simulink model "NAV420_Emulator"  (Simulink 7.3)
settings: Solver=ode45  StartTime=0.0  StopTime=inf  RelTol=1e-3
undefined symbols (not defined in the file or in its folder): serial
libraries: instrumentlib x2
settings Model: Creator=djulzz  LastModifiedBy=djulzz

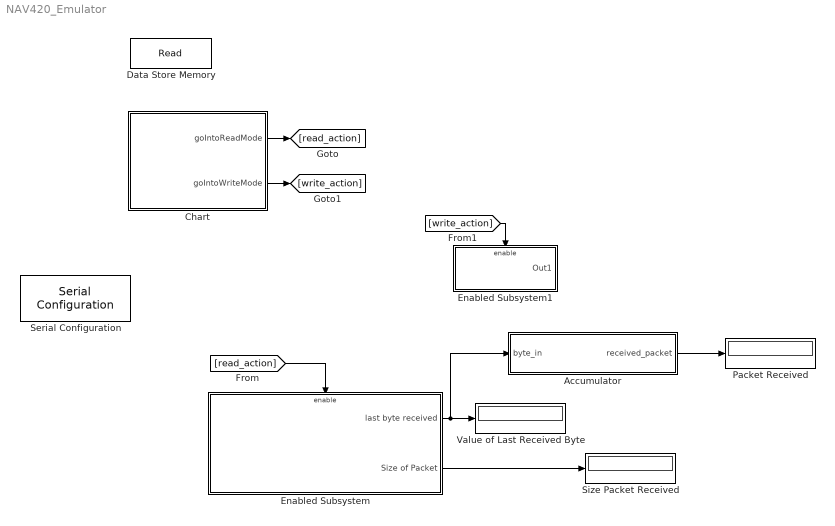
== system NAV420_Emulator ==
  Accumulator : Subsystem
  Chart : Stateflow chart
  Data Store Memory : DataStoreMemory  DataStoreName=Read  ReadBeforeWriteMsg=warning  WriteAfterWriteMsg=warning  WriteAfterReadMsg=warning  InitialValue=1  DataType=double  OutDataType=fixdt(1, 16)  OutScaling=2^0  OutDataTypeStr=double
  Enabled Subsystem : Subsystem  TreatAsAtomicUnit=on
  Enabled Subsystem1 : Subsystem  TreatAsAtomicUnit=on
  Packet Received : Display
  Serial Configuration : instrumentlib/Serial Configuration  Priority=-200000  DialogController=instrumentcreatedialog  DialogControllerArgs=DataTag1  ComPortMenu=COM1  ComPort=COM1  ObjConstructor=serial('COM1');  BaudRate=9600  DataBits=8  Parity=none  StopBits=1  FlowControl=none  Timeout=10  ByteOrder=LittleEndian
  Size Packet Received : Display
  Value of Last Received Byte : Display
  wires:
  Chart/1(goIntoReadMode) -> [read_action]
  Chart/2(goIntoWriteMode) -> [write_action]
  [write_action] -> Enabled Subsystem1/Enable
  Enabled Subsystem/1(last byte received) -> Value of Last Received Byte/1, Accumulator/1(byte_in)
  Enabled Subsystem/2(Size of Packet) -> Size Packet Received/1
  [read_action] -> Enabled Subsystem/Enable
  Accumulator/1(received_packet) -> Packet Received/1

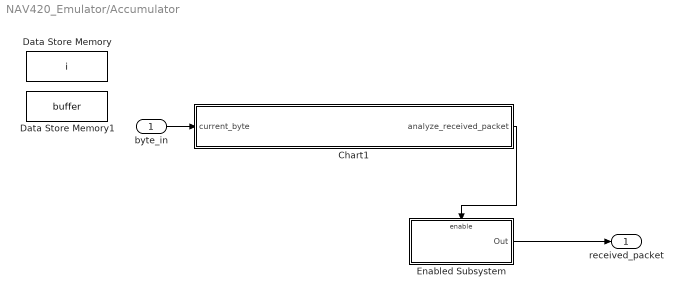
== system NAV420_Emulator/Accumulator ==
  byte_in : Inport  DataType=uint8  OutDataType=fixdt(1, 16)  OutScaling=2^0  OutDataTypeStr=uint8
  Chart1 : Stateflow chart
  Data Store Memory : DataStoreMemory  DataStoreName=i  InitialValue=1  DataType=uint8  OutDataType=fixdt(1, 16)  OutScaling=2^0  OutDataTypeStr=uint8
  Data Store Memory1 : DataStoreMemory  DataStoreName=buffer  InitialValue=1  DataType=uint8  OutDataType=fixdt(1, 16)  OutScaling=2^0  OutDataTypeStr=uint8
  Enabled Subsystem : Subsystem  TreatAsAtomicUnit=on
  received_packet : Outport  DataType=uint8  OutDataType=fixdt(1, 16)  OutScaling=2^0  OutDataTypeStr=uint8
  wires:
  byte_in/1 -> Chart1/1(current_byte)
  Enabled Subsystem/1(Out) -> received_packet/1
  Chart1/1(analyze_received_packet) -> Enabled Subsystem/Enable

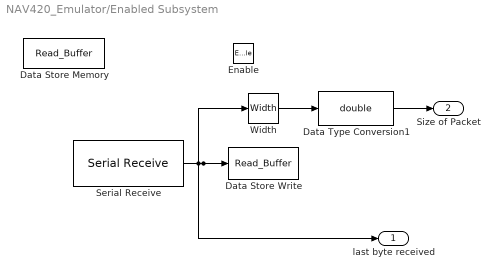
== system NAV420_Emulator/Enabled Subsystem ==
  Enable : EnablePort
  Data Store Memory : DataStoreMemory  DataStoreName=Read_Buffer  InitialValue=1  DataType=uint8  OutDataType=fixdt(1, 16)  OutScaling=2^0  OutDataTypeStr=uint8
  Data Store Write : DataStoreWrite  DataStoreName=Read_Buffer  SampleTime=-1
  Data Type Conversion1 : DataTypeConversion  OutDataTypeMode=double  OutDataType=fixdt(1, 16)  OutScaling=2^0  OutDataTypeStr=double
  Serial Receive : instrumentlib/Serial Receive  DialogController=instrumentcreatedialog  DialogControllerArgs=DataTag0  ComPortMenu=COM1  ComPort=COM1  ObjConstructor=serial('COM1');  Terminator=<none>  DataSize="[1  1]"  DataType=uint8  EnableBlockingMode=on  ActionDataUnavailable=Output last received value  CustomValue=0  SampleTime=0.01
  Width : Width
  last byte received : Outport  DataType=uint8  OutDataType=fixdt(1, 16)  OutScaling=2^0  OutDataTypeStr=uint8
  Size of Packet : Outport  Port=2  DataType=double  OutDataType=fixdt(1, 16)  OutScaling=2^0  OutDataTypeStr=double
  wires:
  Serial Receive/1 -> Data Store Write/1, Width/1, last byte received/1
  Data Type Conversion1/1 -> Size of Packet/1
  Width/1 -> Data Type Conversion1/1

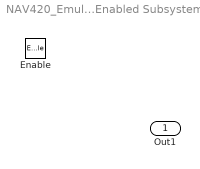
== system NAV420_Emulator/Enabled Subsystem1 ==
  Enable : EnablePort
  Out1 : Outport  OutDataType=fixdt(1, 16)  OutScaling=2^0

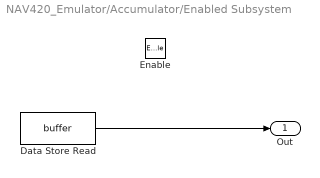
== system NAV420_Emulator/Accumulator/Enabled Subsystem ==
  Enable : EnablePort
  Data Store Read : DataStoreRead  DataStoreName=buffer  SampleTime=0
  Out : Outport  OutDataType=fixdt(1, 16)  OutScaling=2^0
  wires:
  Data Store Read/1 -> Out/1

== stateflow chart Chart ==
  state ReadMode
    goIntoReadMode=1;
  state WriteMode
    goIntoWriteMode=1;
  ReadMode -> WriteMode : [Read==0]
  WriteMode -> ReadMode : [Read==1]
  (default) -> ReadMode
  data: goIntoReadMode output double; goIntoWriteMode output double; Read data_store_memory double

== stateflow chart Accumulator/Chart1 ==
  state First_Byte_of_Packet
    analyze_received_packet=1;
    i=1;
  state First_U
    buffer[1]=current_byte[1];
    i=i++;
  (default) -> First_Byte_of_Packet
  First_Byte_of_Packet -> First_U : [current_byte==85]
  First_U -> First_Byte_of_Packet : [current_byte==85]
  data: current_byte input uint8 size=1; buffer data_store_memory double; i data_store_memory double; analyze_received_packet output double
